simulink model "PMSM_DTC_improved"  (R2014b)
settings: Solver=ode3  StartTime=0.0  StopTime=0.4  FixedStep=5e-6  MaxStep=1e-3  RelTol=1e-4
libraries: powerlib x6, simulink x1
settings Model: Creator=Administrator  LastModifiedBy=Lei
settings SolverCC: SolverResetMethod=Robust
settings DataIOCC: SignalLoggingSaveFormat=ModelDataLogs
settings OptimizationCC: ExpressionDepthLimit=2147483647  InitFltsAndDblsToZero=on
settings DebuggingCC: UnderspecifiedInitializationDetection=Classic  MergeDetectMultiDrivingBlocksExec=none  FcnCallInpInsideContextMsg=UseLocalSettings  StateNameClashWarn=warning
settings GRTTargetCC: CombineOutputUpdateFcns=off  GRTInterface=on

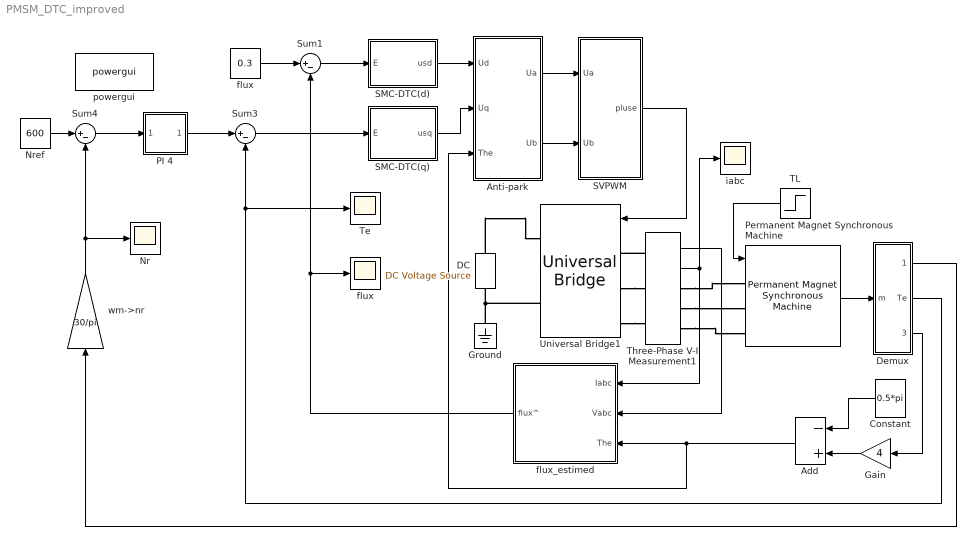
== system PMSM_DTC_improved ==
  Add : Sum  Inputs=-+
  Anti-park : Subsystem
  Constant : Constant  Value=0.5*pi
  DC : powerlib/Electrical Sources/DC Voltage Source  Amplitude=311  Measurements=None
  Demux : Subsystem
  Gain : Gain  Gain=4
  Ground : powerlib/Elements/Ground  LConnTagsString=a
  Nr : Scope
      settings: TickLabels=on  TimeRange=0.3  YMin=575  YMax=605  SaveName=wm  SampleInput=on
  Nref : Constant  Value=600
  PI 4 : Subsystem
      mask Display: disp('PI')
  Permanent Magnet Synchronous Machine : powerlib/Machines/Permanent Magnet Synchronous Machine  NbPhases=3  FluxDistribution=Sinusoidal  RotorType=Salient-pole  MechanicalLoad=Torque Tm  PresetModel=No  ShowDetailedParameters=on  MeasurementBus=off  Resistance=1.2  Inductance=8.5e-3  dqInductances=[8.5e-3,8.5e-3]  La=0.000835  MachineConstant=Torque Constant (N.m / A_peak)  Flux=0.175  VoltageCst=126.966  TorqueCst=1.05  Flat=120  Mechanical=[0.0008 0 4]  PolePairs=4  InitialConditions=[0,0, 0,0]  InitialConditions5ph=[0 0 0 0 0 0]  TsPowergui=0  TsBlock=-1  RefAngle=90 degrees behind phase A axis (modified Park)
  SMC-DTC(d) : Subsystem
  SMC-DTC(q) : Subsystem
  SVPWM : Subsystem
  Sum1 : Sum  Inputs=|+-
  Sum3 : Sum  Inputs=|+-
  Sum4 : Sum  Inputs=|+-
  TL : Step  Time=0.2  After=1.5  SampleTime=0
  Te : Scope
      settings: TickLabels=on  TimeRange=0.35  YMin=1.35  YMax=1.6  SaveName=te  SampleInput=on
  Three-Phase V-I Measurement1 : powerlib/Measurements/Three-Phase V-I Measurement  VoltageMeasurement=phase-to-ground  SetLabelV=off  LabelV=Vabc  Vpu=off  VpuLL=off  CurrentMeasurement=yes  SetLabelI=off  LabelI=Iabc  Ipu=off  Pbase=100e6  Vbase=500e3  OutputType=Complex  PhasorSimulation=off  PSBequivalent=0
  Universal Bridge1 : powerlib/Power Electronics/Universal Bridge  Arms=3  SnubberResistance=1e5  SnubberCapacitance=inf  Device=IGBT / Diodes  Ron=1e-3  Lon=0  ForwardVoltages="[  0  0  ]"  ForwardVoltage=0  GTOparameters=[ 10e-6 , 20e-6 ]  IGBTparameters=[ 1e-6 , 2e-6 ]  Measurements=None  Measurements_2=None  converterType=Rectifier
  flux : Scope
      settings: TickLabels=on  TimeRange=0.4  YMin=0.18  YMax=0.32  SaveName=flux  SampleInput=on
  "flux " : Constant  Value=0.3
  flux_estimed : Subsystem
  iabc : Scope
      settings: TickLabels=on  TimeRange=0.3  YMin=-60  YMax=80  SaveName=iabc  SampleInput=on
  powergui : powerlib/powergui  SimulationMode=Continuous  SolverType=Tustin/Backward Euler (TBE)  SampleTime=50e-6  frequency=60  SPID=off  DisableSnubberDevices=off  DisableRonSwitches=off  DisableVfSwitches=off  SwTol=0  DisplayEquations=off  Interpol=off  methode=off  Ts=0  frequencyindice=0  Pbase=100e6  ErrMax=1e-4  Iterations=50  UnitsV=kV  UnitsW=MW  FunctionMessages=off  echomessages=off  HookPort=off  EnableUseOfTLC=off  x0status=blocks  RestoreLinks=warning  ResistiveCurrentMeasurement=off  Frange=[0:2:500]  Ylog=off  Xlog=on  ShowGrid=off  save=off  variable=ZData  structure=0  ZoomFFT=on  StartTime=0.0  cycles=1  DisplayStyle=1  fundamental=60  FreqAxis=off  MaxFrequency=1000  frequencyindicesteady=1  RmsSteady=1  display=off
  wm->nr : Gain  Gain=30/pi
  wires:
  Anti-park/1(Ua) -> SVPWM/1(Ua)
  Anti-park/2(Ub) -> SVPWM/2(Ub)
  Demux/3(The) -> Gain/1
  SMC-DTC(d)/1(usd) -> Anti-park/1(Ud)
  "flux "/1 -> Sum1/1
  Sum1/1 -> SMC-DTC(d)/1(E)
  SMC-DTC(q)/1(usq) -> Anti-park/2(Uq)
  Permanent Magnet Synchronous Machine/1 -> Demux/1(m)
  Demux/2(Te) -> Te/1, Sum3/2
  Nref/1 -> Sum4/1
  Sum4/1 -> PI 4/1(In1)
  PI 4/1(Out1) -> Sum3/1
  Sum3/1 -> SMC-DTC(q)/1(E)
  wm->nr/1 -> Nr/1, Sum4/2
  TL/1 -> Permanent Magnet Synchronous Machine/1
  SVPWM/1(pluse) -> Universal Bridge1/1
  Demux/1(wm) -> wm->nr/1
  flux_estimed/1(flux^) -> Sum1/2, flux/1
  Three-Phase V-I Measurement1/1 -> flux_estimed/2(Vabc)
  Gain/1 -> Add/2
  Constant/1 -> Add/1
  Add/1 -> Anti-park/3(The), flux_estimed/3(The)
  Three-Phase V-I Measurement1/2 -> flux_estimed/1(Iabc), iabc/1
  connections:
  Ground/LConn1 -- Universal Bridge1/RConn2 -- DC/LConn1
  Three-Phase V-I Measurement1/RConn1 -- Permanent Magnet Synchronous Machine/LConn1
  DC/RConn1 -- Universal Bridge1/RConn1
  Universal Bridge1/LConn2 -- Three-Phase V-I Measurement1/LConn2
  Three-Phase V-I Measurement1/LConn1 -- Universal Bridge1/LConn1
  Universal Bridge1/LConn3 -- Three-Phase V-I Measurement1/LConn3
  Three-Phase V-I Measurement1/RConn3 -- Permanent Magnet Synchronous Machine/LConn3
  Three-Phase V-I Measurement1/RConn2 -- Permanent Magnet Synchronous Machine/LConn2

== system PMSM_DTC_improved/Anti-park ==
  Ud : Inport
  Uq : Inport  Port=2
  The : Inport  Port=3
  Fcn : Fcn  Expr=u(1)*cos(u(3))-u(2)*sin(u(3))
  Fcn1 : Fcn  Expr=u(1)*sin(u(3))+u(2)*cos(u(3))
  Mux1 : Mux  Inputs=3
  Ua : Outport
  Ub : Outport  Port=2
  wires:
  Uq/1 -> Mux1/2
  Ud/1 -> Mux1/1
  Fcn1/1 -> Ub/1
  Fcn/1 -> Ua/1
  Mux1/1 -> Fcn1/1, Fcn/1
  The/1 -> Mux1/3

== system PMSM_DTC_improved/Demux ==
  m : Inport
  Bus Selector1 : BusSelector  OutputSignals=Rotor speed wm (rad/s),Rotor angle thetam (rad),Electromagnetic torque Te (N*m)
  Transfer Fcn : TransferFcn  Numerator=[7000]  Denominator=[1 7000]
  wm : Outport
  Te : Outport  Port=2
  The : Outport  Port=3
  wires:
  m/1 -> Bus Selector1/1
  Bus Selector1/1 -> wm/1  "<Rotor speed wm (rad/s)>"
  Bus Selector1/2 -> The/1  "<Rotor angle thetam (rad)>"
  Bus Selector1/3 -> Transfer Fcn/1  "<Electromagnetic torque Te (N*m)>"
  Transfer Fcn/1 -> Te/1

== system PMSM_DTC_improved/PI 4 ==
  In1 : Inport
  Add : Sum
  Gain : Gain  Gain=0.05
  Gain1 : Gain  Gain=20
  Integrator : Integrator
  Saturation : Saturate  UpperLimit=50  LowerLimit=-50
  Out1 : Outport
  wires:
  Gain1/1 -> Integrator/1
  In1/1 -> Gain/1, Gain1/1
  Gain/1 -> Add/1
  Integrator/1 -> Add/2
  Add/1 -> Saturation/1
  Saturation/1 -> Out1/1

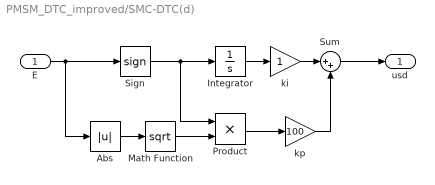
== system PMSM_DTC_improved/SMC-DTC(d) ==
  E : Inport
  Abs : Abs
  Integrator : Integrator
  Math Function : Math  Operator=sqrt  SaturateOnIntegerOverflow=on
  Product : Product  RndMeth=Zero
  Sign : Signum
  Sum : Sum  Inputs=|++
  ki : Gain
  kp : Gain  Gain=100
  usd : Outport
  wires:
  Sum/1 -> usd/1
  E/1 -> Sign/1, Abs/1
  Sign/1 -> Integrator/1, Product/1
  Integrator/1 -> ki/1
  Abs/1 -> Math Function/1
  Math Function/1 -> Product/2
  Product/1 -> kp/1
  kp/1 -> Sum/2
  ki/1 -> Sum/1

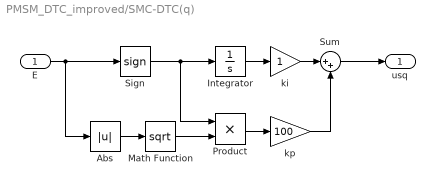
== system PMSM_DTC_improved/SMC-DTC(q) ==
  E : Inport
  Abs : Abs
  Integrator : Integrator
  Math Function : Math  Operator=sqrt  SaturateOnIntegerOverflow=on
  Product : Product  RndMeth=Zero
  Sign : Signum
  Sum : Sum  Inputs=|++
  ki : Gain
  kp : Gain  Gain=100
  usq : Outport
  wires:
  ki/1 -> Sum/1
  kp/1 -> Sum/2
  Product/1 -> kp/1
  Math Function/1 -> Product/2
  Abs/1 -> Math Function/1
  Integrator/1 -> ki/1
  Sign/1 -> Product/1, Integrator/1
  E/1 -> Abs/1, Sign/1
  Sum/1 -> usq/1

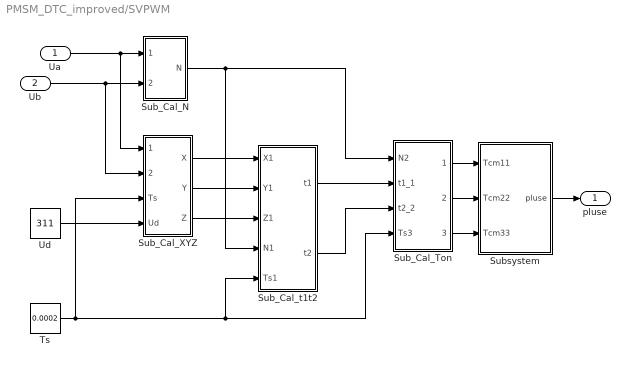
== system PMSM_DTC_improved/SVPWM ==
  Ua : Inport
  Ub : Inport  Port=2
  Sub_Cal_N : Subsystem
  Sub_Cal_Ton : Subsystem
  Sub_Cal_XYZ : Subsystem
  Sub_Cal_t1t2 : Subsystem
  Subsystem : Subsystem
  Ts : Constant  Value=0.0002
  Ud : Constant  Value=311
  pluse : Outport
  wires:
  Ua/1 -> Sub_Cal_N/1(Ualfa), Sub_Cal_XYZ/1(Ualfa1)
  Ub/1 -> Sub_Cal_N/2(Ubeta), Sub_Cal_XYZ/2(Ubeta1)
  Sub_Cal_XYZ/1(X) -> Sub_Cal_t1t2/1(X1)
  Sub_Cal_XYZ/2(Y) -> Sub_Cal_t1t2/2(Y1)
  Sub_Cal_XYZ/3(Z) -> Sub_Cal_t1t2/3(Z1)
  Sub_Cal_t1t2/1(t1) -> Sub_Cal_Ton/2(t1_1)
  Sub_Cal_Ton/1(Tcm1) -> Subsystem/1(Tcm11)
  Sub_Cal_Ton/2(Tcm2) -> Subsystem/2(Tcm22)
  Ts/1 -> Sub_Cal_Ton/4(Ts3), Sub_Cal_t1t2/5(Ts1), Sub_Cal_XYZ/3(Ts)
  Sub_Cal_Ton/3(Tcm3) -> Subsystem/3(Tcm33)
  Subsystem/1(pluse) -> pluse/1
  Sub_Cal_t1t2/2(t2) -> Sub_Cal_Ton/3(t2_2)
  Ud/1 -> Sub_Cal_XYZ/4(Ud)
  Sub_Cal_N/1(N) -> Sub_Cal_Ton/1(N2), Sub_Cal_t1t2/4(N1)

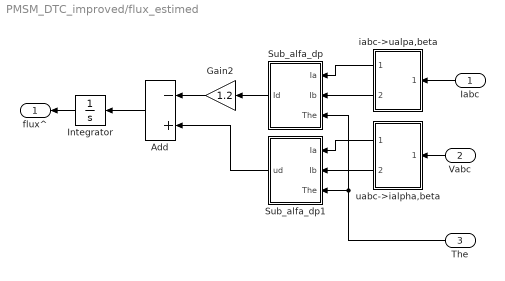
== system PMSM_DTC_improved/flux_estimed ==
  Iabc : Inport
  Vabc : Inport  Port=2
  The : Inport  Port=3
  Add : Sum  Inputs=-+
  Gain2 : Gain  Gain=1.2
  Integrator : Integrator
  Sub_alfa_dp : Subsystem
  Sub_alfa_dp1 : Subsystem
  iabc->ualpa,beta : Subsystem
  uabc->ialpha,beta : Subsystem
  flux^ : Outport
  wires:
  iabc->ualpa,beta/1(ialfa) -> Sub_alfa_dp/1(Ia)
  iabc->ualpa,beta/2(ibeta) -> Sub_alfa_dp/2(Ib)
  uabc->ialpha,beta/1(ualfa) -> Sub_alfa_dp1/1(Ia)
  uabc->ialpha,beta/2(ubeta) -> Sub_alfa_dp1/2(Ib)
  Sub_alfa_dp1/1(ud) -> Add/2
  Sub_alfa_dp/1(Id) -> Gain2/1
  Gain2/1 -> Add/1
  Add/1 -> Integrator/1
  Iabc/1 -> iabc->ualpa,beta/1(iabc)
  Integrator/1 -> flux^/1
  Vabc/1 -> uabc->ialpha,beta/1(uabc)
  The/1 -> Sub_alfa_dp1/3(The), Sub_alfa_dp/3(The)

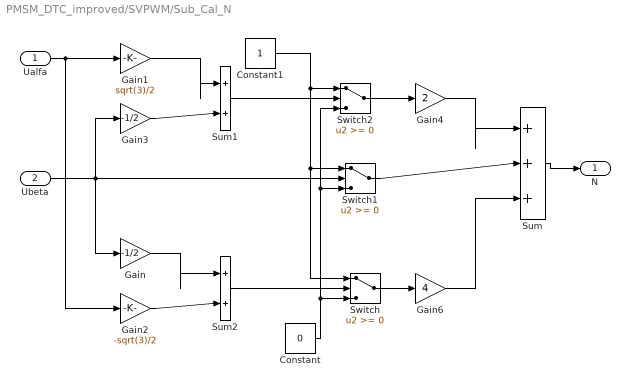
== system PMSM_DTC_improved/SVPWM/Sub_Cal_N ==
  Ualfa : Inport
  Ubeta : Inport  Port=2
  Constant : Constant  Value=0
  Constant1 : Constant
  Gain : Gain  Gain=-1/2
  Gain1 : Gain  Gain=sqrt(3)/2
  Gain2 : Gain  Gain=-sqrt(3)/2
  Gain3 : Gain  Gain=-1/2
  Gain4 : Gain  Gain=2
  Gain6 : Gain  Gain=4
  Sum : Sum  Inputs=|+++
  Sum1 : Sum  Inputs=|++
  Sum2 : Sum  Inputs=|++
  Switch : Switch
  Switch1 : Switch
  Switch2 : Switch
  N : Outport
  wires:
  Ubeta/1 -> Switch1/2, Gain3/1, Gain/1
  Gain1/1 -> Sum1/1
  Gain3/1 -> Sum1/2
  Sum1/1 -> Switch2/2
  Ualfa/1 -> Gain1/1, Gain2/1
  Gain/1 -> Sum2/1
  Gain2/1 -> Sum2/2
  Sum2/1 -> Switch/2
  Constant1/1 -> Switch/1, Switch1/1, Switch2/1
  Constant/1 -> Switch2/3, Switch1/3, Switch/3
  Switch/1 -> Gain6/1
  Switch2/1 -> Gain4/1
  Gain4/1 -> Sum/1
  Switch1/1 -> Sum/2
  Gain6/1 -> Sum/3
  Sum/1 -> N/1

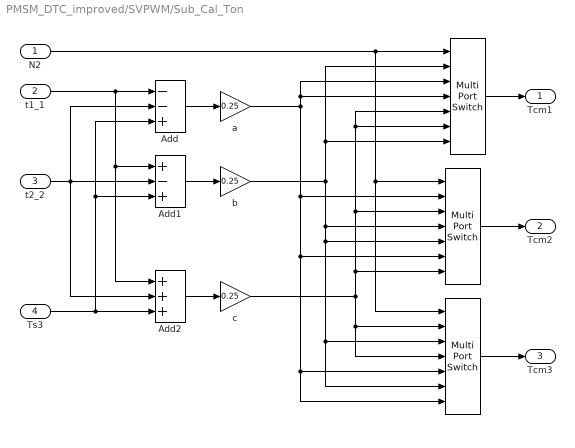
== system PMSM_DTC_improved/SVPWM/Sub_Cal_Ton ==
  N2 : Inport
  t1_1 : Inport  Port=2
  t2_2 : Inport  Port=3
  Ts3 : Inport  Port=4
  " " : MultiPortSwitch  Inputs=6
  "  " : MultiPortSwitch  Inputs=6
  "    " : MultiPortSwitch  Inputs=6
  Add : Sum  Inputs=--+
  Add1 : Sum  Inputs=+-+
  Add2 : Sum  Inputs=+++
  a : Gain  Gain=0.25
  b : Gain  Gain=0.25
  c : Gain  Gain=0.25
  Tcm1 : Outport
  Tcm2 : Outport  Port=2
  Tcm3 : Outport  Port=3
  wires:
  N2/1 -> "  "/1, " "/1, "    "/1
  t1_1/1 -> Add/1, Add1/1, Add2/1
  t2_2/1 -> Add/2, Add1/2, Add2/2
  Ts3/1 -> Add/3, Add1/3, Add2/3
  Add/1 -> a/1
  Add1/1 -> b/1
  Add2/1 -> c/1
  "  "/1 -> Tcm1/1
  " "/1 -> Tcm2/1
  "    "/1 -> Tcm3/1
  b/1 -> "  "/7, "  "/2, " "/4, " "/5, "    "/3, "    "/6
  a/1 -> " "/2, " "/6, "    "/5, "    "/7, "  "/4, "  "/3
  c/1 -> "  "/5, "  "/6, " "/3, " "/7, "    "/2, "    "/4

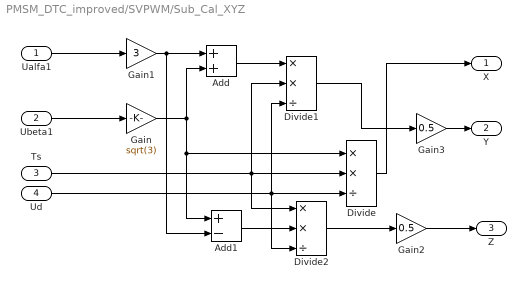
== system PMSM_DTC_improved/SVPWM/Sub_Cal_XYZ ==
  Ualfa1 : Inport
  Ubeta1 : Inport  Port=2
  Ts : Inport  Port=3
  Ud : Inport  Port=4
  Add : Sum
  Add1 : Sum  Inputs=+-
  Divide : Product  Inputs=**/
  Divide1 : Product  Inputs=**/
  Divide2 : Product  Inputs=**/
  Gain : Gain  Gain=sqrt(3)
  Gain1 : Gain  Gain=3
  Gain2 : Gain  Gain=0.5
  Gain3 : Gain  Gain=0.5
  X : Outport
  Y : Outport  Port=2
  Z : Outport  Port=3
  wires:
  Ubeta1/1 -> Gain/1
  Gain/1 -> Add/2, Divide/1, Add1/1
  Ts/1 -> Divide/2, Divide1/2, Divide2/1
  Ud/1 -> Divide/3, Divide1/3, Divide2/3
  Ualfa1/1 -> Gain1/1
  Gain1/1 -> Add/1, Add1/2
  Add/1 -> Divide1/1
  Add1/1 -> Divide2/2
  Divide2/1 -> Gain2/1
  Gain2/1 -> Z/1
  Divide/1 -> X/1
  Divide1/1 -> Gain3/1
  Gain3/1 -> Y/1

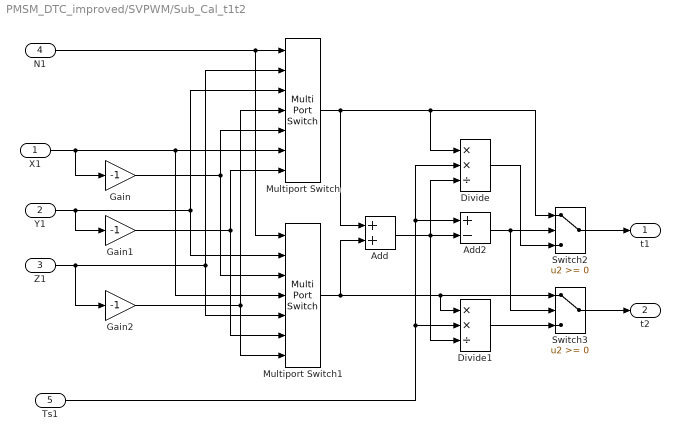
== system PMSM_DTC_improved/SVPWM/Sub_Cal_t1t2 ==
  X1 : Inport
  Y1 : Inport  Port=2
  Z1 : Inport  Port=3
  N1 : Inport  Port=4
  Ts1 : Inport  Port=5
  Add : Sum
  Add2 : Sum  Inputs=+-
  Divide : Product  Inputs=**/
  Divide1 : Product  Inputs=**/
  Gain : Gain  Gain=-1
  Gain1 : Gain  Gain=-1
  Gain2 : Gain  Gain=-1
  Multiport Switch : MultiPortSwitch  Inputs=6
  Multiport Switch1 : MultiPortSwitch  Inputs=6
  Switch2 : Switch
  Switch3 : Switch
  t1 : Outport
  t2 : Outport  Port=2
  wires:
  N1/1 -> Multiport Switch/1, Multiport Switch1/1
  Y1/1 -> Gain1/1, Multiport Switch/3, Multiport Switch1/2
  X1/1 -> Gain/1, Multiport Switch/6, Multiport Switch1/4
  Z1/1 -> Gain2/1, Multiport Switch/2, Multiport Switch1/5
  Multiport Switch/1 -> Add/1, Divide/1, Switch2/1
  Multiport Switch1/1 -> Add/2, Switch3/1, Divide1/1
  Ts1/1 -> Divide1/2, Divide/2, Add2/1
  Add2/1 -> Switch2/2, Switch3/2
  Divide/1 -> Switch2/3
  Divide1/1 -> Switch3/3
  Switch3/1 -> t2/1
  Switch2/1 -> t1/1
  Add/1 -> Divide/3, Divide1/3, Add2/2
  Gain1/1 -> Multiport Switch1/6, Multiport Switch/7
  Gain2/1 -> Multiport Switch/4, Multiport Switch1/7
  Gain/1 -> Multiport Switch/5, Multiport Switch1/3

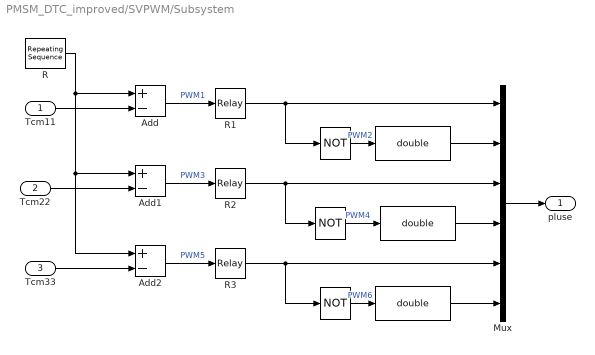
== system PMSM_DTC_improved/SVPWM/Subsystem ==
  Tcm11 : Inport
  Tcm22 : Inport  Port=2
  Tcm33 : Inport  Port=3
  " " : Logic  Operator=NOT  AllPortsSameDT=off  OutDataTypeStr=boolean
  "  " : DataTypeConversion  OutDataTypeStr=double
  "   " : Logic  Operator=NOT  AllPortsSameDT=off  OutDataTypeStr=boolean
  "     " : DataTypeConversion  OutDataTypeStr=double
  "       " : Logic  Operator=NOT  AllPortsSameDT=off  OutDataTypeStr=boolean
  "         " : DataTypeConversion  OutDataTypeStr=double
  Add : Sum  Inputs=+-
  Add1 : Sum  Inputs=+-
  Add2 : Sum  Inputs=+-
  Mux : Mux  Inputs=6
  R : simulink/Sources/Repeating Sequence  rep_seq_t="[0  0.0001  0.0002]"  rep_seq_y="[0  0.0001  0]"
  R1 : Relay
  R2 : Relay
  R3 : Relay
  pluse : Outport
  wires:
  "  "/1 -> Mux/2
  "     "/1 -> Mux/4
  "         "/1 -> Mux/6
  R2/1 -> Mux/3, "   "/1
  R3/1 -> Mux/5, "       "/1
  R1/1 -> Mux/1, " "/1
  Mux/1 -> pluse/1
  "       "/1 -> "         "/1  "PWM6"
  "   "/1 -> "     "/1  "PWM4"
  " "/1 -> "  "/1  "PWM2"
  Add2/1 -> R3/1  "PWM5"
  Add1/1 -> R2/1  "PWM3"
  Add/1 -> R1/1  "PWM1"
  R/1 -> Add/1, Add1/1, Add2/1
  Tcm33/1 -> Add2/2
  Tcm22/1 -> Add1/2
  Tcm11/1 -> Add/2

== system PMSM_DTC_improved/flux_estimed/Sub_alfa_dp ==
  Ia : Inport
  Ib : Inport  Port=2
  The : Inport  Port=3
  Fcn : Fcn  Expr=cos(u)
  Fcn1 : Fcn  Expr=sin(u)
  Fcn2 : Fcn  Expr=u(1)*u(3)+u(2)*u(4)
  Mux : Mux
  Id : Outport
  wires:
  The/1 -> Fcn/1, Fcn1/1
  Ia/1 -> Mux/1
  Ib/1 -> Mux/2
  Fcn/1 -> Mux/3
  Fcn1/1 -> Mux/4
  Mux/1 -> Fcn2/1
  Fcn2/1 -> Id/1

== system PMSM_DTC_improved/flux_estimed/Sub_alfa_dp1 ==
  Ia : Inport
  Ib : Inport  Port=2
  The : Inport  Port=3
  Fcn : Fcn  Expr=cos(u)
  Fcn1 : Fcn  Expr=sin(u)
  Fcn2 : Fcn  Expr=u(1)*u(3)+u(2)*u(4)
  Mux : Mux
  ud : Outport
  wires:
  Fcn2/1 -> ud/1
  Mux/1 -> Fcn2/1
  Fcn1/1 -> Mux/4
  Fcn/1 -> Mux/3
  Ib/1 -> Mux/2
  Ia/1 -> Mux/1
  The/1 -> Fcn1/1, Fcn/1

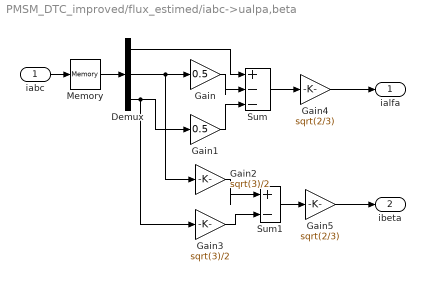
== system PMSM_DTC_improved/flux_estimed/iabc->ualpa,beta ==
  iabc : Inport
  Demux : Demux  Outputs=3
  Gain : Gain  Gain=0.5
  Gain1 : Gain  Gain=0.5
  Gain2 : Gain  Gain=sqrt(3)/2
  Gain3 : Gain  Gain=sqrt(3)/2
  Gain4 : Gain  Gain=sqrt(2/3)
  Gain5 : Gain  Gain=sqrt(2/3)
  Memory : Memory
  Sum : Sum  Inputs=|+--
  Sum1 : Sum  Inputs=|+-
  ialfa : Outport
  ibeta : Outport  Port=2
  wires:
  iabc/1 -> Memory/1
  Demux/2 -> Gain/1, Gain2/1
  Sum/1 -> Gain4/1
  Sum1/1 -> Gain5/1
  Demux/1 -> Sum/1
  Demux/3 -> Gain1/1, Gain3/1
  Gain2/1 -> Sum1/1
  Gain3/1 -> Sum1/2
  Gain/1 -> Sum/2
  Gain1/1 -> Sum/3
  Gain4/1 -> ialfa/1
  Gain5/1 -> ibeta/1
  Memory/1 -> Demux/1

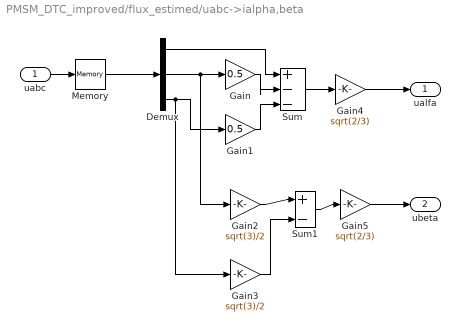
== system PMSM_DTC_improved/flux_estimed/uabc->ialpha,beta ==
  uabc : Inport
  Demux : Demux  Outputs=3
  Gain : Gain  Gain=0.5
  Gain1 : Gain  Gain=0.5
  Gain2 : Gain  Gain=sqrt(3)/2
  Gain3 : Gain  Gain=sqrt(3)/2
  Gain4 : Gain  Gain=sqrt(2/3)
  Gain5 : Gain  Gain=sqrt(2/3)
  Memory : Memory
  Sum : Sum  Inputs=|+--
  Sum1 : Sum  Inputs=|+-
  ualfa : Outport
  ubeta : Outport  Port=2
  wires:
  uabc/1 -> Memory/1
  Demux/2 -> Gain/1, Gain2/1
  Sum/1 -> Gain4/1
  Sum1/1 -> Gain5/1
  Demux/1 -> Sum/1
  Demux/3 -> Gain1/1, Gain3/1
  Gain2/1 -> Sum1/1
  Gain3/1 -> Sum1/2
  Gain/1 -> Sum/2
  Gain1/1 -> Sum/3
  Gain4/1 -> ualfa/1
  Gain5/1 -> ubeta/1
  Memory/1 -> Demux/1
